simulink library "LWS"  (R2024a)
settings: Solver=VariableStepAuto  StartTime=0.0  StopTime=10.0  RelTol=1e-3
undefined symbols (not defined in the file or in its folder): raptor_xcp_function, StateCAN
libraries: Utilities x4, Raptor_lib x2, simulink x1
settings Model: Creator=hyuga  LastModifiedBy=hyuga
settings ConfigComp: CovBoundaryAbsTol=1.0e-5

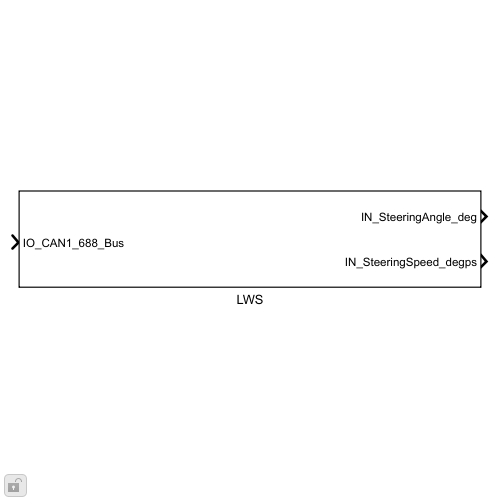
[thumbnail: Simulink's stored preview of the top-level diagram]
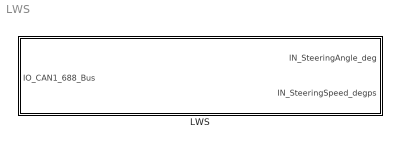
== system LWS ==
  LWS : Subsystem

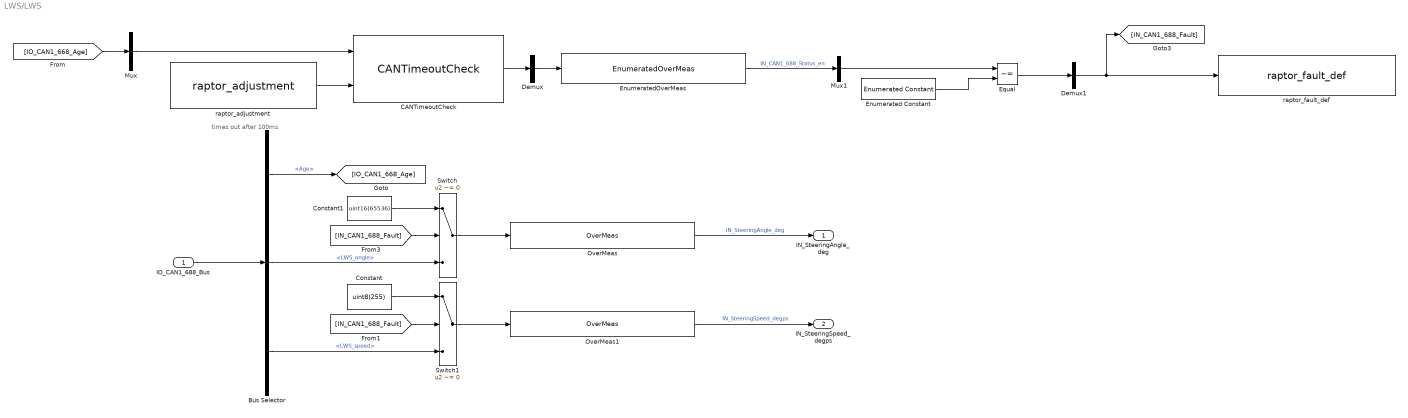
== system LWS/LWS ==
  note: times out after 100ms
  IO_CAN1_688_Bus : Inport
  Bus Selector : BusSelector  OutputSignals=Age,LWS_angle,LWS_speed
  CANTimeoutCheck : Utilities/CANTimeoutCheck
  Constant : Constant  Value=uint8(255)
  Constant1 : Constant  Value=uint16(65536)
  Demux : Demux  Outputs=1
  Demux1 : Demux  Outputs=1
  Enumerated Constant : simulink/Sources/Enumerated Constant  OutDataTypeStr=Enum: StateCAN  Value=StateCAN.Normal  SampleTime=inf
  EnumeratedOverMeas : Utilities/EnumeratedOverMeas  sigName='IN_CAN1_688_Status_en'  enumName='StateCAN'
  Equal : RelationalOperator  Operator=~=  OutDataTypeStr=boolean  RndMeth=Simplest  InputSameDT=off
  Mux : Mux  Inputs=1
  Mux1 : Mux  Inputs=1
  OverMeas : Utilities/OverMeas  sigName='IN_SteeringAngle_deg'  minimum=-inf  maximum=inf
  OverMeas1 : Utilities/OverMeas  sigName='IN_SteeringSpeed_degps'  minimum=-inf  maximum=inf
  Switch : Switch  Criteria=u2 ~= 0  SaturateOnIntegerOverflow=off  InputSameDT=off
  Switch1 : Switch  Criteria=u2 ~= 0  SaturateOnIntegerOverflow=off  InputSameDT=off
  raptor_adjustment : Raptor_lib/Data Storage/raptor_adjustment  paramName='IN_LWS_na'  nameSource=Parameter  initValue=20  dataType=uint32  storage=Calibration  calDispType=Number  calEnum={'False', 'True'}  calGain=1.0  calOffset=0.0  calMax=inf  calMin=-inf  calFormat='-1'  calUnit=''  calHelp=''  calAccess=1  calFunction=raptor_xcp_function(gcb)  calDispHeaders=off  calColHeaders={'Col1' 'Col2' 'Col3'}  calRowHeaders={'Row1' 'Row2' 'Row3'}
      settings: SourceProductName=Raptor
  raptor_fault_def : Raptor_lib/Faults/raptor_fault_def  faultName='IN_CAN1_688_Fault'  persist=on  sticky=off  emisRelated=off  permanent=off  singleTrip=off  clearMethod=Standard  xLimit=25  yLimit=50  calEnable=on  addDisable=off  calAccess=1  calFunction='System | FaultManager'
      settings: SourceProductName=Raptor
  IN_SteeringAngle_deg : Outport
  IN_SteeringSpeed_degps : Outport  Port=2
  wires:
  Constant/1 -> Switch1/1
  Constant1/1 -> Switch/1
  [IN_CAN1_688_Fault] -> Switch1/2
  OverMeas1/1 -> IN_SteeringSpeed_degps/1  "IN_SteeringSpeed_degps"
  OverMeas/1 -> IN_SteeringAngle_deg/1  "IN_SteeringAngle_deg"
  Switch/1 -> OverMeas/1
  Switch1/1 -> OverMeas1/1
  Bus Selector/3 -> Switch1/3  "<LWS_speed>"
  Bus Selector/2 -> Switch/3  "<LWS_angle>"
  [IN_CAN1_688_Fault] -> Switch/2
  Bus Selector/1 -> [IO_CAN1_668_Age]  "<Age>"
  Equal/1 -> Demux1/1
  Mux1/1 -> Equal/1
  Enumerated Constant/1 -> Equal/2
  EnumeratedOverMeas/1 -> Mux1/1  "IN_CAN1_688_Status_en"
  [IO_CAN1_668_Age] -> Mux/1
  Demux1/1 -> raptor_fault_def/1, [IN_CAN1_688_Fault]
  CANTimeoutCheck/1 -> Demux/1
  raptor_adjustment/1 -> CANTimeoutCheck/2
  Mux/1 -> CANTimeoutCheck/1
  Demux/1 -> EnumeratedOverMeas/1
  IO_CAN1_688_Bus/1 -> Bus Selector/1
